simulink model "HANcoder_E407_TTA_Group2"  (R2018b)
settings: Solver=FixedStepDiscrete  StartTime=0.0  StopTime=1  FixedStep=0.01  RelTol=1e-3
PreLoadFcn:
  | librarySetup
  | eval([bdroot,'_startup']) %Calling [modelName]_startup.m
values from neighbouring files (symbols this model uses):
  BackUp_Role = 4    [HANcoder_E407_TTA_Group2_startup.m]
  basic_cycle_duration_bc0 = TM_Reset_Board   + COMP_duration    (= 550)    [HANcoder_E407_TTA_Group2_startup.m]    (also in HANcoder_E407_TTA_Template_startup.m = 212)
  basic_cycle_duration_bc1 = TM_Reset_Var_bc1 + COMP_duration    (= 610)    [HANcoder_E407_TTA_Group2_startup.m]    (also in HANcoder_E407_TTA_Template_startup.m = 212)
  board1_online = Simulink.Parameter    [HANcoder_E407_TTA_Group2_startup.m]
  board2_online = Simulink.Parameter    [HANcoder_E407_TTA_Group2_startup.m]
  board3_online = Simulink.Parameter    [HANcoder_E407_TTA_Group2_startup.m]
  board4_online = Simulink.Parameter    [HANcoder_E407_TTA_Group2_startup.m]
  comm_delay_estimation1 = round(comm_delay_measured1*hardware_granularity/frequency_IRQ)    [HANcoder_E407_TTA_Group2_startup.m]    (also in HANcoder_E407_TTA_Template_startup.m)
  comm_delay_estimation2 = round(comm_delay_measured2*hardware_granularity/frequency_IRQ)    [HANcoder_E407_TTA_Group2_startup.m]    (also in HANcoder_E407_TTA_Template_startup.m)
  COMM_Period = 50    [HANcoder_E407_TTA_Group2_startup.m]    (also in HANcoder_E407_TTA_Template_startup.m = 40)
  COMM_Phase1 = Simulink.Parameter    [HANcoder_E407_TTA_Group2_startup.m]    (also in HANcoder_E407_TTA_Template_startup.m)
  COMM_Phase2 = Simulink.Parameter    [HANcoder_E407_TTA_Group2_startup.m]    (also in HANcoder_E407_TTA_Template_startup.m)
  COMM_Phase_init1 = Simulink.Parameter    [HANcoder_E407_TTA_Group2_startup.m]    (also in HANcoder_E407_TTA_Template_startup.m)
  COMM_Phase_init2 = Simulink.Parameter    [HANcoder_E407_TTA_Group2_startup.m]    (also in HANcoder_E407_TTA_Template_startup.m)
  COMP_duration = 20    [HANcoder_E407_TTA_Group2_startup.m]    (also in HANcoder_E407_TTA_Template_startup.m = 4)
  Controller1_Board = 1    [HANcoder_E407_TTA_Group2_startup.m]    (also in HANcoder_E407_TTA_Template_startup.m)
  Controller2_Board = 2    [HANcoder_E407_TTA_Group2_startup.m]    (also in HANcoder_E407_TTA_Template_startup.m)
  Controller3_Board = 3    [HANcoder_E407_TTA_Group2_startup.m]    (also in HANcoder_E407_TTA_Template_startup.m)
  Controller4_Board = 4    [HANcoder_E407_TTA_Group2_startup.m]
  delta_a_set = Simulink.Parameter    [HANcoder_E407_TTA_Group2_startup.m]
  delta_f_set = Simulink.Parameter    [HANcoder_E407_TTA_Group2_startup.m]
  delta_max = 1    [HANcoder_E407_TTA_Group2_startup.m]
  delta_min = -1    [HANcoder_E407_TTA_Group2_startup.m]
  delta_precision = 6    [HANcoder_E407_TTA_Group2_startup.m]
  e_width = 0.1    [HANcoder_E407_TTA_Group2_startup.m]
  ErrorLog_ID = 31    [HANcoder_E407_TTA_Group2_startup.m]
  frequency_IRQ = 100    [HANcoder_E407_TTA_Group2_startup.m]    (also in HANcoder_E407_TTA_Template_startup.m)
  HANtuneOverride = Simulink.Parameter    [HANcoder_E407_TTA_Group2_startup.m]    (also in HANcoder_E407_TTA_Template_startup.m)
  hardware_granularity = 1000000    [HANcoder_E407_TTA_Group2_startup.m]    (also in HANcoder_E407_TTA_Template_startup.m)
  I_a = 2.25    [HANcoder_E407_TTA_Group2_startup.m]
  I_f = 2.25    [HANcoder_E407_TTA_Group2_startup.m]
  idle_time_init = basic_cycle_duration_bc0 + basic_cycle_duration_bc1    (= 1160)    [HANcoder_E407_TTA_Group2_startup.m]    (also in HANcoder_E407_TTA_Template_startup.m = 424)
  Input_Gen_Board = 5    [HANcoder_E407_TTA_Group2_startup.m]
  LA_Clock_Gr = 1    [HANcoder_E407_TTA_Group2_startup.m]    (also in HANcoder_E407_TTA_Template_startup.m)
  LA_COMM_dly = 1    [HANcoder_E407_TTA_Group2_startup.m]    (also in HANcoder_E407_TTA_Template_startup.m)
  LA_COMM_Err = 1    [HANcoder_E407_TTA_Group2_startup.m]    (also in HANcoder_E407_TTA_Template_startup.m)
  LA_E_Desync = 1    [HANcoder_E407_TTA_Group2_startup.m]    (also in HANcoder_E407_TTA_Template_startup.m)
  LA_MEX_Flag = 1    [HANcoder_E407_TTA_Group2_startup.m]    (also in HANcoder_E407_TTA_Template_startup.m)
  LA_Task_Act = 1    [HANcoder_E407_TTA_Group2_startup.m]    (also in HANcoder_E407_TTA_Template_startup.m)
  m_v = 100.0    (= 100)    [HANcoder_E407_TTA_Group2_startup.m]
  Master_Role = 1    [HANcoder_E407_TTA_Group2_startup.m]    (also in HANcoder_E407_TTA_Template_startup.m)
  matrix_cycle_duration = basic_cycle_duration_bc0 + basic_cycle_duration_bc1    (= 1160)    [HANcoder_E407_TTA_Group2_startup.m]    (also in HANcoder_E407_TTA_Template_startup.m = 424)
  matrix_rows = 2    [HANcoder_E407_TTA_Group2_startup.m]    (also in HANcoder_E407_TTA_Template_startup.m)
  max_desync = 15    [HANcoder_E407_TTA_Group2_startup.m]    (also in HANcoder_E407_TTA_Template_startup.m)
  max_num_msgs_CAN1 = 2^Tx_bit_number-1    (= 7)    [HANcoder_E407_TTA_Group2_startup.m]    (also in HANcoder_E407_TTA_Template_startup.m)
  max_num_msgs_CAN2 = max_num_msgs_CAN1    (= 7)    [HANcoder_E407_TTA_Group2_startup.m]    (also in HANcoder_E407_TTA_Template_startup.m)
  min_desync = (-1)*max_desync    (= -15)    [HANcoder_E407_TTA_Group2_startup.m]    (also in HANcoder_E407_TTA_Template_startup.m)
  OutControl1_ID = 23    [HANcoder_E407_TTA_Group2_startup.m]    (also in HANcoder_E407_TTA_Template_startup.m)
  OutControl2_ID = 24    [HANcoder_E407_TTA_Group2_startup.m]    (also in HANcoder_E407_TTA_Template_startup.m)
  OutEmulator_ID = 25    [HANcoder_E407_TTA_Group2_startup.m]    (also in HANcoder_E407_TTA_Template_startup.m)
  R_al = 0.10    (= 0.1)    [HANcoder_E407_TTA_Group2_startup.m]
  R_ar = 0.10    (= 0.1)    [HANcoder_E407_TTA_Group2_startup.m]
  R_fl = 0.10    (= 0.1)    [HANcoder_E407_TTA_Group2_startup.m]
  R_fr = 0.10    (= 0.1)    [HANcoder_E407_TTA_Group2_startup.m]
  script_run = Simulink.Parameter    [HANcoder_E407_TTA_Group2_startup.m]    (also in HANcoder_E407_TTA_Template_startup.m)
  SensorValues_ID = 22    [HANcoder_E407_TTA_Group2_startup.m]    (also in HANcoder_E407_TTA_Template_startup.m)
  SetValues_ID = 21    [HANcoder_E407_TTA_Group2_startup.m]    (also in HANcoder_E407_TTA_Template_startup.m)
  Slave_Role = 3    [HANcoder_E407_TTA_Group2_startup.m]    (also in HANcoder_E407_TTA_Template_startup.m = 2)
  speed_k_d = Simulink.Parameter    [HANcoder_E407_TTA_Group2_startup.m]
  speed_k_i = Simulink.Parameter    [HANcoder_E407_TTA_Group2_startup.m]
  speed_k_p = Simulink.Parameter    [HANcoder_E407_TTA_Group2_startup.m]
  speed_max = 10    [HANcoder_E407_TTA_Group2_startup.m]
  speed_min = -10    [HANcoder_E407_TTA_Group2_startup.m]
  speed_precision = 3    [HANcoder_E407_TTA_Group2_startup.m]
  Sync_ID = 1    [HANcoder_E407_TTA_Group2_startup.m]    (also in HANcoder_E407_TTA_Template_startup.m)
  tau_max = 5    [HANcoder_E407_TTA_Group2_startup.m]
  tau_min = -5    [HANcoder_E407_TTA_Group2_startup.m]
  tau_range = abs(tau_max) + abs(tau_min)    [HANcoder_E407_TTA_Group2_startup.m]
  theta_max = (speed_max/R_fr)*matrix_cycle_duration*frequency_IRQ/hardware_granularity    (= 11.6)    [HANcoder_E407_TTA_Group2_startup.m]
  theta_min = (-1)*theta_max    (= -11.6)    [HANcoder_E407_TTA_Group2_startup.m]
  theta_precision = 7-(fix(log2(theta_max))+1)    [HANcoder_E407_TTA_Group2_startup.m]
  Tl_a = 0.6    [HANcoder_E407_TTA_Group2_startup.m]
  Tl_f = 0.6    [HANcoder_E407_TTA_Group2_startup.m]
  TM_bc0_1 = basic_cycle_start    (= 0)    [HANcoder_E407_TTA_Group2_startup.m]
  TM_bc0_10 = TM_bc0_9 + COMP_duration    (= 270)    [HANcoder_E407_TTA_Group2_startup.m]
  TM_bc0_11 = TM_bc0_10 + COMP_duration    (= 290)    [HANcoder_E407_TTA_Group2_startup.m]
  TM_bc0_12 = TM_bc0_11  + COMM_duration    (= 340)    [HANcoder_E407_TTA_Group2_startup.m]
  TM_bc0_13 = TM_bc0_12 + COMP_duration    (= 360)    [HANcoder_E407_TTA_Group2_startup.m]
  TM_bc0_14 = TM_bc0_13 + COMP_duration    (= 380)    [HANcoder_E407_TTA_Group2_startup.m]
  TM_bc0_15 = TM_bc0_14  + COMM_duration    (= 430)    [HANcoder_E407_TTA_Group2_startup.m]
  TM_bc0_16 = TM_bc0_15 + COMP_duration    (= 450)    [HANcoder_E407_TTA_Group2_startup.m]
  TM_bc0_17 = TM_bc0_16 + COMP_duration    (= 470)    [HANcoder_E407_TTA_Group2_startup.m]
  TM_bc0_18 = TM_bc0_17 + COMP_duration    (= 490)    [HANcoder_E407_TTA_Group2_startup.m]
  TM_bc0_2 = TM_bc0_1   + COMM_duration    (= 50)    [HANcoder_E407_TTA_Group2_startup.m]
  TM_bc0_3 = TM_bc0_2  + COMP_duration    (= 70)    [HANcoder_E407_TTA_Group2_startup.m]
  TM_bc0_3_2 = TM_bc0_3   + 2    (= 72)    [HANcoder_E407_TTA_Group2_startup.m]
  TM_bc0_4 = TM_bc0_3   + COMP_duration    (= 90)    [HANcoder_E407_TTA_Group2_startup.m]
  TM_bc0_4_2 = TM_bc0_4    + 2    (= 92)    [HANcoder_E407_TTA_Group2_startup.m]
  TM_bc0_5 = TM_bc0_4    + COMP_duration    (= 110)    [HANcoder_E407_TTA_Group2_startup.m]
  TM_bc0_6 = TM_bc0_5  + COMM_duration    (= 160)    [HANcoder_E407_TTA_Group2_startup.m]
  TM_bc0_7 = TM_bc0_6 + COMP_duration    (= 180)    [HANcoder_E407_TTA_Group2_startup.m]
  TM_bc0_8 = TM_bc0_7 + COMP_duration    (= 200)    [HANcoder_E407_TTA_Group2_startup.m]
  TM_bc0_9 = TM_bc0_8  + COMM_duration    (= 250)    [HANcoder_E407_TTA_Group2_startup.m]
  TM_bc0_9_2 = TM_bc0_9 + 2    (= 252)    [HANcoder_E407_TTA_Group2_startup.m]
  TM_bc1_18 = TM_Check_Output_Emulator + COMP_duration    (= 520)    [HANcoder_E407_TTA_Group2_startup.m]
  TM_bc1_19 = TM_bc1_18 + COMM_duration    (= 570)    [HANcoder_E407_TTA_Group2_startup.m]
  TM_bc1_19_2 = TM_bc1_19 + 2    (= 572)    [HANcoder_E407_TTA_Group2_startup.m]
  TM_Check_Output_Control1 = TM_COMM_Output_Control1 + COMP_duration    (= 340)    [HANcoder_E407_TTA_Group2_startup.m]
  TM_Check_Output_Control2 = TM_COMM_Output_Control2 + COMM_duration    (= 410)    [HANcoder_E407_TTA_Group2_startup.m]
  TM_Check_Output_Emulator = TM_COMM_Output_Emulator + COMM_duration    (= 500)    [HANcoder_E407_TTA_Group2_startup.m]
  TM_Check_Output_Emulator_2 = TM_Check_Output_Emulator + 2    (= 502)    [HANcoder_E407_TTA_Group2_startup.m]
  TM_Check_Sensor_Values = TM_COMM_Sensor_Values + COMM_duration    (= 210)    [HANcoder_E407_TTA_Group2_startup.m]
  TM_Check_Sensor_Values_2 = TM_Check_Sensor_Values + 2    (= 212)    [HANcoder_E407_TTA_Group2_startup.m]
  TM_Check_Set_Values = TM_COMM_Set_Values + COMM_duration    (= 140)    [HANcoder_E407_TTA_Group2_startup.m]
  TM_Check_Set_Values_2 = TM_Check_Set_Values + 2    (= 142)    [HANcoder_E407_TTA_Group2_startup.m]
  TM_COMM_Output_Control1 = TM_Velocity + COMM_duration    (= 320)    [HANcoder_E407_TTA_Group2_startup.m]
  TM_COMM_Output_Control2 = TM_Check_Output_Control1 + COMP_duration    (= 360)    [HANcoder_E407_TTA_Group2_startup.m]
  TM_COMM_Output_Emulator = TM_TMR + COMP_duration    (= 450)    [HANcoder_E407_TTA_Group2_startup.m]
  TM_COMM_Sensor_Values = TM_Check_Set_Values + COMP_duration    (= 160)    [HANcoder_E407_TTA_Group2_startup.m]
  TM_COMM_Set_Values = TM_bc0_3 + COMP_duration    (= 90)    [HANcoder_E407_TTA_Group2_startup.m]
  TM_COMM_Sync = basic_cycle_start    (= 0)    [HANcoder_E407_TTA_Group2_startup.m]    (also in HANcoder_E407_TTA_Template_startup.m)
  TM_Data_bc0 = TM_COMM_Sync    (= 0)    [HANcoder_E407_TTA_Group2_startup.m]    (also in HANcoder_E407_TTA_Template_startup.m)
  TM_Data_bc1 = TM_Data_bc0(1:4)    [HANcoder_E407_TTA_Group2_startup.m]    (also in HANcoder_E407_TTA_Template_startup.m)
  TM_Reset_Board = TM_Reset_Var   + COMP_duration    (= 530)    [HANcoder_E407_TTA_Group2_startup.m]    (also in HANcoder_E407_TTA_Template_startup.m = 208)
  TM_Reset_Var = TM_bc0_18  + COMP_duration    (= 510)    [HANcoder_E407_TTA_Group2_startup.m]    (also in HANcoder_E407_TTA_Template_startup.m = 204)
  TM_Reset_Var_bc1 = TM_bc1_19 + COMP_duration    (= 590)    [HANcoder_E407_TTA_Group2_startup.m]    (also in HANcoder_E407_TTA_Template_startup.m = 200)
  TM_Reset_Var_bc1_2 = TM_Reset_Var_bc1 + 2    (= 592)    [HANcoder_E407_TTA_Group2_startup.m]    (also in HANcoder_E407_TTA_Template_startup.m = 202)
  TM_Steer = TM_Check_Sensor_Values + COMP_duration    (= 230)    [HANcoder_E407_TTA_Group2_startup.m]
  TM_TMR = TM_Check_Output_Control2 + COMP_duration    (= 430)    [HANcoder_E407_TTA_Group2_startup.m]
  TM_TMR_2 = TM_TMR + 1    (= 431)    [HANcoder_E407_TTA_Group2_startup.m]
  ... (+19 more)
undefined symbols (not defined in the file or in its folder): A0, A1, A2, A3, A4, CON2, CON4, D10, D12, D13, D8, D9
libraries: hdlsllib x340, HANcoder_STM32_Target x28, simulink x5, simulink_extras x1
(part 6 of 36)

== system HANcoder_E407_TTA_Group2/HANcoder STM32 Target - E407-STM32 algorithm/TTA CAN System/CAN1 Recieve/RxID_CAN/SetValues_ID_CAN/CAN receive1 ==
  In1 : Inport
  Enabled Subsystem : Subsystem  TreatAsAtomicUnit=on
  S-Function : M-S-Function  FunctionName=sfcn_can_receive  Parameters=tsamp, canBus, outputNumber, dataType, byteOrder
  Out1 : Outport
  Out2 : Outport  Port=2
  Out3 : Outport  Port=3
  Out4 : Outport  Port=4
  Out5 : Outport  Port=5
  Out6 : Outport  Port=6
  Out7 : Outport  Port=7
  Out8 : Outport  Port=8
  Out9 : Outport  Port=9
  wires:
  S-Function/9 -> Enabled Subsystem/8(In8)
  S-Function/4 -> Enabled Subsystem/3(In3)
  S-Function/5 -> Enabled Subsystem/4(In4)
  S-Function/8 -> Enabled Subsystem/7(In7)
  S-Function/7 -> Enabled Subsystem/6(In6)
  S-Function/6 -> Enabled Subsystem/5(In5)
  Enabled Subsystem/8(Out8) -> Out9/1
  Enabled Subsystem/7(Out7) -> Out8/1
  Enabled Subsystem/6(Out6) -> Out7/1
  Enabled Subsystem/5(Out5) -> Out6/1
  Enabled Subsystem/4(Out4) -> Out5/1
  Enabled Subsystem/3(Out3) -> Out4/1
  Enabled Subsystem/2(Out2) -> Out3/1
  Enabled Subsystem/1(Out1) -> Out2/1
  S-Function/3 -> Enabled Subsystem/2(In2)
  S-Function/2 -> Enabled Subsystem/1(In1)
  S-Function/1 -> Out1/1, Enabled Subsystem/Enable
  In1/1 -> S-Function/1

== system HANcoder_E407_TTA_Group2/HANcoder STM32 Target - E407-STM32 algorithm/TTA CAN System/CAN1 Recieve/RxID_CAN/Sync_ID_CAN/CAN receive1 ==
  In1 : Inport
  Enabled Subsystem : Subsystem  TreatAsAtomicUnit=on
  S-Function : M-S-Function  FunctionName=sfcn_can_receive  Parameters=tsamp, canBus, outputNumber, dataType, byteOrder
  Out1 : Outport
  Out2 : Outport  Port=2
  Out3 : Outport  Port=3
  Out4 : Outport  Port=4
  Out5 : Outport  Port=5
  Out6 : Outport  Port=6
  Out7 : Outport  Port=7
  Out8 : Outport  Port=8
  Out9 : Outport  Port=9
  wires:
  S-Function/9 -> Enabled Subsystem/8(In8)
  S-Function/4 -> Enabled Subsystem/3(In3)
  S-Function/5 -> Enabled Subsystem/4(In4)
  S-Function/8 -> Enabled Subsystem/7(In7)
  S-Function/7 -> Enabled Subsystem/6(In6)
  S-Function/6 -> Enabled Subsystem/5(In5)
  Enabled Subsystem/8(Out8) -> Out9/1
  Enabled Subsystem/7(Out7) -> Out8/1
  Enabled Subsystem/6(Out6) -> Out7/1
  Enabled Subsystem/5(Out5) -> Out6/1
  Enabled Subsystem/4(Out4) -> Out5/1
  Enabled Subsystem/3(Out3) -> Out4/1
  Enabled Subsystem/2(Out2) -> Out3/1
  Enabled Subsystem/1(Out1) -> Out2/1
  S-Function/3 -> Enabled Subsystem/2(In2)
  S-Function/2 -> Enabled Subsystem/1(In1)
  S-Function/1 -> Out1/1, Enabled Subsystem/Enable
  In1/1 -> S-Function/1

== system HANcoder_E407_TTA_Group2/HANcoder STM32 Target - E407-STM32 algorithm/TTA CAN System/CAN1 Recieve/RxID_CAN/Vote1_ID_CAN/CAN receive1 ==
  In1 : Inport
  Enabled Subsystem : Subsystem  TreatAsAtomicUnit=on
  S-Function : M-S-Function  FunctionName=sfcn_can_receive  Parameters=tsamp, canBus, outputNumber, dataType, byteOrder
  Out1 : Outport
  Out2 : Outport  Port=2
  Out3 : Outport  Port=3
  Out4 : Outport  Port=4
  Out5 : Outport  Port=5
  Out6 : Outport  Port=6
  Out7 : Outport  Port=7
  Out8 : Outport  Port=8
  Out9 : Outport  Port=9
  wires:
  In1/1 -> S-Function/1
  S-Function/1 -> Enabled Subsystem/Enable, Out1/1
  S-Function/2 -> Enabled Subsystem/1(In1)
  S-Function/3 -> Enabled Subsystem/2(In2)
  Enabled Subsystem/1(Out1) -> Out2/1
  Enabled Subsystem/2(Out2) -> Out3/1
  Enabled Subsystem/3(Out3) -> Out4/1
  Enabled Subsystem/4(Out4) -> Out5/1
  Enabled Subsystem/5(Out5) -> Out6/1
  Enabled Subsystem/6(Out6) -> Out7/1
  Enabled Subsystem/7(Out7) -> Out8/1
  Enabled Subsystem/8(Out8) -> Out9/1
  S-Function/6 -> Enabled Subsystem/5(In5)
  S-Function/7 -> Enabled Subsystem/6(In6)
  S-Function/8 -> Enabled Subsystem/7(In7)
  S-Function/5 -> Enabled Subsystem/4(In4)
  S-Function/4 -> Enabled Subsystem/3(In3)
  S-Function/9 -> Enabled Subsystem/8(In8)

== system HANcoder_E407_TTA_Group2/HANcoder STM32 Target - E407-STM32 algorithm/TTA CAN System/CAN1 Recieve/RxID_CAN/Vote2_ID_CAN/CAN receive1 ==
  In1 : Inport
  Enabled Subsystem : Subsystem  TreatAsAtomicUnit=on
  S-Function : M-S-Function  FunctionName=sfcn_can_receive  Parameters=tsamp, canBus, outputNumber, dataType, byteOrder
  Out1 : Outport
  Out2 : Outport  Port=2
  Out3 : Outport  Port=3
  Out4 : Outport  Port=4
  Out5 : Outport  Port=5
  Out6 : Outport  Port=6
  Out7 : Outport  Port=7
  Out8 : Outport  Port=8
  Out9 : Outport  Port=9
  wires:
  In1/1 -> S-Function/1
  S-Function/1 -> Enabled Subsystem/Enable, Out1/1
  S-Function/2 -> Enabled Subsystem/1(In1)
  S-Function/3 -> Enabled Subsystem/2(In2)
  Enabled Subsystem/1(Out1) -> Out2/1
  Enabled Subsystem/2(Out2) -> Out3/1
  Enabled Subsystem/3(Out3) -> Out4/1
  Enabled Subsystem/4(Out4) -> Out5/1
  Enabled Subsystem/5(Out5) -> Out6/1
  Enabled Subsystem/6(Out6) -> Out7/1
  Enabled Subsystem/7(Out7) -> Out8/1
  Enabled Subsystem/8(Out8) -> Out9/1
  S-Function/6 -> Enabled Subsystem/5(In5)
  S-Function/7 -> Enabled Subsystem/6(In6)
  S-Function/8 -> Enabled Subsystem/7(In7)
  S-Function/5 -> Enabled Subsystem/4(In4)
  S-Function/4 -> Enabled Subsystem/3(In3)
  S-Function/9 -> Enabled Subsystem/8(In8)

== system HANcoder_E407_TTA_Group2/HANcoder STM32 Target - E407-STM32 algorithm/TTA CAN System/CAN1 Recieve/RxID_CAN/Vote3_ID_CAN/CAN receive1 ==
  In1 : Inport
  Enabled Subsystem : Subsystem  TreatAsAtomicUnit=on
  S-Function : M-S-Function  FunctionName=sfcn_can_receive  Parameters=tsamp, canBus, outputNumber, dataType, byteOrder
  Out1 : Outport
  Out2 : Outport  Port=2
  Out3 : Outport  Port=3
  Out4 : Outport  Port=4
  Out5 : Outport  Port=5
  Out6 : Outport  Port=6
  Out7 : Outport  Port=7
  Out8 : Outport  Port=8
  Out9 : Outport  Port=9
  wires:
  In1/1 -> S-Function/1
  S-Function/1 -> Enabled Subsystem/Enable, Out1/1
  S-Function/2 -> Enabled Subsystem/1(In1)
  S-Function/3 -> Enabled Subsystem/2(In2)
  Enabled Subsystem/1(Out1) -> Out2/1
  Enabled Subsystem/2(Out2) -> Out3/1
  Enabled Subsystem/3(Out3) -> Out4/1
  Enabled Subsystem/4(Out4) -> Out5/1
  Enabled Subsystem/5(Out5) -> Out6/1
  Enabled Subsystem/6(Out6) -> Out7/1
  Enabled Subsystem/7(Out7) -> Out8/1
  Enabled Subsystem/8(Out8) -> Out9/1
  S-Function/6 -> Enabled Subsystem/5(In5)
  S-Function/7 -> Enabled Subsystem/6(In6)
  S-Function/8 -> Enabled Subsystem/7(In7)
  S-Function/5 -> Enabled Subsystem/4(In4)
  S-Function/4 -> Enabled Subsystem/3(In3)
  S-Function/9 -> Enabled Subsystem/8(In8)

== system HANcoder_E407_TTA_Group2/HANcoder STM32 Target - E407-STM32 algorithm/TTA CAN System/CAN1 Recieve/RxID_CAN/Vote4_ID_CAN1/CAN receive1 ==
  In1 : Inport
  Enabled Subsystem : Subsystem  TreatAsAtomicUnit=on
  S-Function : M-S-Function  FunctionName=sfcn_can_receive  Parameters=tsamp, canBus, outputNumber, dataType, byteOrder
  Out1 : Outport
  Out2 : Outport  Port=2
  Out3 : Outport  Port=3
  Out4 : Outport  Port=4
  Out5 : Outport  Port=5
  Out6 : Outport  Port=6
  Out7 : Outport  Port=7
  Out8 : Outport  Port=8
  Out9 : Outport  Port=9
  wires:
  In1/1 -> S-Function/1
  S-Function/1 -> Enabled Subsystem/Enable, Out1/1
  S-Function/2 -> Enabled Subsystem/1(In1)
  S-Function/3 -> Enabled Subsystem/2(In2)
  Enabled Subsystem/1(Out1) -> Out2/1
  Enabled Subsystem/2(Out2) -> Out3/1
  Enabled Subsystem/3(Out3) -> Out4/1
  Enabled Subsystem/4(Out4) -> Out5/1
  Enabled Subsystem/5(Out5) -> Out6/1
  Enabled Subsystem/6(Out6) -> Out7/1
  Enabled Subsystem/7(Out7) -> Out8/1
  Enabled Subsystem/8(Out8) -> Out9/1
  S-Function/6 -> Enabled Subsystem/5(In5)
  S-Function/7 -> Enabled Subsystem/6(In6)
  S-Function/8 -> Enabled Subsystem/7(In7)
  S-Function/5 -> Enabled Subsystem/4(In4)
  S-Function/4 -> Enabled Subsystem/3(In3)
  S-Function/9 -> Enabled Subsystem/8(In8)

== system HANcoder_E407_TTA_Group2/HANcoder STM32 Target - E407-STM32 algorithm/TTA CAN System/CAN2 Recieve/RxID_CAN/OutControl1_ID_CAN/CAN receive1 ==
  In1 : Inport
  Enabled Subsystem : Subsystem  TreatAsAtomicUnit=on
  S-Function : M-S-Function  FunctionName=sfcn_can_receive  Parameters=tsamp, canBus, outputNumber, dataType, byteOrder
  Out1 : Outport
  Out2 : Outport  Port=2
  Out3 : Outport  Port=3
  Out4 : Outport  Port=4
  Out5 : Outport  Port=5
  Out6 : Outport  Port=6
  Out7 : Outport  Port=7
  Out8 : Outport  Port=8
  Out9 : Outport  Port=9
  wires:
  S-Function/9 -> Enabled Subsystem/8(In8)
  S-Function/4 -> Enabled Subsystem/3(In3)
  S-Function/5 -> Enabled Subsystem/4(In4)
  S-Function/8 -> Enabled Subsystem/7(In7)
  S-Function/7 -> Enabled Subsystem/6(In6)
  S-Function/6 -> Enabled Subsystem/5(In5)
  Enabled Subsystem/8(Out8) -> Out9/1
  Enabled Subsystem/7(Out7) -> Out8/1
  Enabled Subsystem/6(Out6) -> Out7/1
  Enabled Subsystem/5(Out5) -> Out6/1
  Enabled Subsystem/4(Out4) -> Out5/1
  Enabled Subsystem/3(Out3) -> Out4/1
  Enabled Subsystem/2(Out2) -> Out3/1
  Enabled Subsystem/1(Out1) -> Out2/1
  S-Function/3 -> Enabled Subsystem/2(In2)
  S-Function/2 -> Enabled Subsystem/1(In1)
  S-Function/1 -> Out1/1, Enabled Subsystem/Enable
  In1/1 -> S-Function/1

== system HANcoder_E407_TTA_Group2/HANcoder STM32 Target - E407-STM32 algorithm/TTA CAN System/CAN2 Recieve/RxID_CAN/OutControl2_ID_CAN/CAN receive1 ==
  In1 : Inport
  Enabled Subsystem : Subsystem  TreatAsAtomicUnit=on
  S-Function : M-S-Function  FunctionName=sfcn_can_receive  Parameters=tsamp, canBus, outputNumber, dataType, byteOrder
  Out1 : Outport
  Out2 : Outport  Port=2
  Out3 : Outport  Port=3
  Out4 : Outport  Port=4
  Out5 : Outport  Port=5
  Out6 : Outport  Port=6
  Out7 : Outport  Port=7
  Out8 : Outport  Port=8
  Out9 : Outport  Port=9
  wires:
  In1/1 -> S-Function/1
  S-Function/1 -> Enabled Subsystem/Enable, Out1/1
  S-Function/2 -> Enabled Subsystem/1(In1)
  S-Function/3 -> Enabled Subsystem/2(In2)
  Enabled Subsystem/1(Out1) -> Out2/1
  Enabled Subsystem/2(Out2) -> Out3/1
  Enabled Subsystem/3(Out3) -> Out4/1
  Enabled Subsystem/4(Out4) -> Out5/1
  Enabled Subsystem/5(Out5) -> Out6/1
  Enabled Subsystem/6(Out6) -> Out7/1
  Enabled Subsystem/7(Out7) -> Out8/1
  Enabled Subsystem/8(Out8) -> Out9/1
  S-Function/6 -> Enabled Subsystem/5(In5)
  S-Function/7 -> Enabled Subsystem/6(In6)
  S-Function/8 -> Enabled Subsystem/7(In7)
  S-Function/5 -> Enabled Subsystem/4(In4)
  S-Function/4 -> Enabled Subsystem/3(In3)
  S-Function/9 -> Enabled Subsystem/8(In8)

== system HANcoder_E407_TTA_Group2/HANcoder STM32 Target - E407-STM32 algorithm/TTA CAN System/CAN2 Recieve/RxID_CAN/OutEmulator_ID_CAN/CAN receive1 ==
  In1 : Inport
  Enabled Subsystem : Subsystem  TreatAsAtomicUnit=on
  S-Function : M-S-Function  FunctionName=sfcn_can_receive  Parameters=tsamp, canBus, outputNumber, dataType, byteOrder
  Out1 : Outport
  Out2 : Outport  Port=2
  Out3 : Outport  Port=3
  Out4 : Outport  Port=4
  Out5 : Outport  Port=5
  Out6 : Outport  Port=6
  Out7 : Outport  Port=7
  Out8 : Outport  Port=8
  Out9 : Outport  Port=9
  wires:
  S-Function/9 -> Enabled Subsystem/8(In8)
  S-Function/4 -> Enabled Subsystem/3(In3)
  S-Function/5 -> Enabled Subsystem/4(In4)
  S-Function/8 -> Enabled Subsystem/7(In7)
  S-Function/7 -> Enabled Subsystem/6(In6)
  S-Function/6 -> Enabled Subsystem/5(In5)
  Enabled Subsystem/8(Out8) -> Out9/1
  Enabled Subsystem/7(Out7) -> Out8/1
  Enabled Subsystem/6(Out6) -> Out7/1
  Enabled Subsystem/5(Out5) -> Out6/1
  Enabled Subsystem/4(Out4) -> Out5/1
  Enabled Subsystem/3(Out3) -> Out4/1
  Enabled Subsystem/2(Out2) -> Out3/1
  Enabled Subsystem/1(Out1) -> Out2/1
  S-Function/3 -> Enabled Subsystem/2(In2)
  S-Function/2 -> Enabled Subsystem/1(In1)
  S-Function/1 -> Out1/1, Enabled Subsystem/Enable
  In1/1 -> S-Function/1

== system HANcoder_E407_TTA_Group2/HANcoder STM32 Target - E407-STM32 algorithm/TTA CAN System/CAN2 Recieve/RxID_CAN/OutEmulator_ID_CAN1/CAN receive1 ==
  In1 : Inport
  Enabled Subsystem : Subsystem  TreatAsAtomicUnit=on
  S-Function : M-S-Function  FunctionName=sfcn_can_receive  Parameters=tsamp, canBus, outputNumber, dataType, byteOrder
  Out1 : Outport
  Out2 : Outport  Port=2
  Out3 : Outport  Port=3
  Out4 : Outport  Port=4
  Out5 : Outport  Port=5
  Out6 : Outport  Port=6
  Out7 : Outport  Port=7
  Out8 : Outport  Port=8
  Out9 : Outport  Port=9
  wires:
  S-Function/9 -> Enabled Subsystem/8(In8)
  S-Function/4 -> Enabled Subsystem/3(In3)
  S-Function/5 -> Enabled Subsystem/4(In4)
  S-Function/8 -> Enabled Subsystem/7(In7)
  S-Function/7 -> Enabled Subsystem/6(In6)
  S-Function/6 -> Enabled Subsystem/5(In5)
  Enabled Subsystem/8(Out8) -> Out9/1
  Enabled Subsystem/7(Out7) -> Out8/1
  Enabled Subsystem/6(Out6) -> Out7/1
  Enabled Subsystem/5(Out5) -> Out6/1
  Enabled Subsystem/4(Out4) -> Out5/1
  Enabled Subsystem/3(Out3) -> Out4/1
  Enabled Subsystem/2(Out2) -> Out3/1
  Enabled Subsystem/1(Out1) -> Out2/1
  S-Function/3 -> Enabled Subsystem/2(In2)
  S-Function/2 -> Enabled Subsystem/1(In1)
  S-Function/1 -> Out1/1, Enabled Subsystem/Enable
  In1/1 -> S-Function/1

== system HANcoder_E407_TTA_Group2/HANcoder STM32 Target - E407-STM32 algorithm/TTA CAN System/CAN2 Recieve/RxID_CAN/SensorValues_ID_CAN/CAN receive1 ==
  In1 : Inport
  Enabled Subsystem : Subsystem  TreatAsAtomicUnit=on
  S-Function : M-S-Function  FunctionName=sfcn_can_receive  Parameters=tsamp, canBus, outputNumber, dataType, byteOrder
  Out1 : Outport
  Out2 : Outport  Port=2
  Out3 : Outport  Port=3
  Out4 : Outport  Port=4
  Out5 : Outport  Port=5
  Out6 : Outport  Port=6
  Out7 : Outport  Port=7
  Out8 : Outport  Port=8
  Out9 : Outport  Port=9
  wires:
  In1/1 -> S-Function/1
  S-Function/1 -> Enabled Subsystem/Enable, Out1/1
  S-Function/2 -> Enabled Subsystem/1(In1)
  S-Function/3 -> Enabled Subsystem/2(In2)
  Enabled Subsystem/1(Out1) -> Out2/1
  Enabled Subsystem/2(Out2) -> Out3/1
  Enabled Subsystem/3(Out3) -> Out4/1
  Enabled Subsystem/4(Out4) -> Out5/1
  Enabled Subsystem/5(Out5) -> Out6/1
  Enabled Subsystem/6(Out6) -> Out7/1
  Enabled Subsystem/7(Out7) -> Out8/1
  Enabled Subsystem/8(Out8) -> Out9/1
  S-Function/6 -> Enabled Subsystem/5(In5)
  S-Function/7 -> Enabled Subsystem/6(In6)
  S-Function/8 -> Enabled Subsystem/7(In7)
  S-Function/5 -> Enabled Subsystem/4(In4)
  S-Function/4 -> Enabled Subsystem/3(In3)
  S-Function/9 -> Enabled Subsystem/8(In8)

== system HANcoder_E407_TTA_Group2/HANcoder STM32 Target - E407-STM32 algorithm/TTA CAN System/CAN2 Recieve/RxID_CAN/SetValues_ID_CAN/CAN receive1 ==
  In1 : Inport
  Enabled Subsystem : Subsystem  TreatAsAtomicUnit=on
  S-Function : M-S-Function  FunctionName=sfcn_can_receive  Parameters=tsamp, canBus, outputNumber, dataType, byteOrder
  Out1 : Outport
  Out2 : Outport  Port=2
  Out3 : Outport  Port=3
  Out4 : Outport  Port=4
  Out5 : Outport  Port=5
  Out6 : Outport  Port=6
  Out7 : Outport  Port=7
  Out8 : Outport  Port=8
  Out9 : Outport  Port=9
  wires:
  S-Function/9 -> Enabled Subsystem/8(In8)
  S-Function/4 -> Enabled Subsystem/3(In3)
  S-Function/5 -> Enabled Subsystem/4(In4)
  S-Function/8 -> Enabled Subsystem/7(In7)
  S-Function/7 -> Enabled Subsystem/6(In6)
  S-Function/6 -> Enabled Subsystem/5(In5)
  Enabled Subsystem/8(Out8) -> Out9/1
  Enabled Subsystem/7(Out7) -> Out8/1
  Enabled Subsystem/6(Out6) -> Out7/1
  Enabled Subsystem/5(Out5) -> Out6/1
  Enabled Subsystem/4(Out4) -> Out5/1
  Enabled Subsystem/3(Out3) -> Out4/1
  Enabled Subsystem/2(Out2) -> Out3/1
  Enabled Subsystem/1(Out1) -> Out2/1
  S-Function/3 -> Enabled Subsystem/2(In2)
  S-Function/2 -> Enabled Subsystem/1(In1)
  S-Function/1 -> Out1/1, Enabled Subsystem/Enable
  In1/1 -> S-Function/1

== system HANcoder_E407_TTA_Group2/HANcoder STM32 Target - E407-STM32 algorithm/TTA CAN System/CAN2 Recieve/RxID_CAN/Sync_ID_CAN/CAN receive1 ==
  In1 : Inport
  Enabled Subsystem : Subsystem  TreatAsAtomicUnit=on
  S-Function : M-S-Function  FunctionName=sfcn_can_receive  Parameters=tsamp, canBus, outputNumber, dataType, byteOrder
  Out1 : Outport
  Out2 : Outport  Port=2
  Out3 : Outport  Port=3
  Out4 : Outport  Port=4
  Out5 : Outport  Port=5
  Out6 : Outport  Port=6
  Out7 : Outport  Port=7
  Out8 : Outport  Port=8
  Out9 : Outport  Port=9
  wires:
  S-Function/9 -> Enabled Subsystem/8(In8)
  S-Function/4 -> Enabled Subsystem/3(In3)
  S-Function/5 -> Enabled Subsystem/4(In4)
  S-Function/8 -> Enabled Subsystem/7(In7)
  S-Function/7 -> Enabled Subsystem/6(In6)
  S-Function/6 -> Enabled Subsystem/5(In5)
  Enabled Subsystem/8(Out8) -> Out9/1
  Enabled Subsystem/7(Out7) -> Out8/1
  Enabled Subsystem/6(Out6) -> Out7/1
  Enabled Subsystem/5(Out5) -> Out6/1
  Enabled Subsystem/4(Out4) -> Out5/1
  Enabled Subsystem/3(Out3) -> Out4/1
  Enabled Subsystem/2(Out2) -> Out3/1
  Enabled Subsystem/1(Out1) -> Out2/1
  S-Function/3 -> Enabled Subsystem/2(In2)
  S-Function/2 -> Enabled Subsystem/1(In1)
  S-Function/1 -> Out1/1, Enabled Subsystem/Enable
  In1/1 -> S-Function/1

== system HANcoder_E407_TTA_Group2/HANcoder STM32 Target - E407-STM32 algorithm/TTA CAN System/CAN2 Recieve/RxID_CAN/Vote1_ID_CAN/CAN receive1 ==
  In1 : Inport
  Enabled Subsystem : Subsystem  TreatAsAtomicUnit=on
  S-Function : M-S-Function  FunctionName=sfcn_can_receive  Parameters=tsamp, canBus, outputNumber, dataType, byteOrder
  Out1 : Outport
  Out2 : Outport  Port=2
  Out3 : Outport  Port=3
  Out4 : Outport  Port=4
  Out5 : Outport  Port=5
  Out6 : Outport  Port=6
  Out7 : Outport  Port=7
  Out8 : Outport  Port=8
  Out9 : Outport  Port=9
  wires:
  In1/1 -> S-Function/1
  S-Function/1 -> Enabled Subsystem/Enable, Out1/1
  S-Function/2 -> Enabled Subsystem/1(In1)
  S-Function/3 -> Enabled Subsystem/2(In2)
  Enabled Subsystem/1(Out1) -> Out2/1
  Enabled Subsystem/2(Out2) -> Out3/1
  Enabled Subsystem/3(Out3) -> Out4/1
  Enabled Subsystem/4(Out4) -> Out5/1
  Enabled Subsystem/5(Out5) -> Out6/1
  Enabled Subsystem/6(Out6) -> Out7/1
  Enabled Subsystem/7(Out7) -> Out8/1
  Enabled Subsystem/8(Out8) -> Out9/1
  S-Function/6 -> Enabled Subsystem/5(In5)
  S-Function/7 -> Enabled Subsystem/6(In6)
  S-Function/8 -> Enabled Subsystem/7(In7)
  S-Function/5 -> Enabled Subsystem/4(In4)
  S-Function/4 -> Enabled Subsystem/3(In3)
  S-Function/9 -> Enabled Subsystem/8(In8)

== system HANcoder_E407_TTA_Group2/HANcoder STM32 Target - E407-STM32 algorithm/TTA CAN System/CAN2 Recieve/RxID_CAN/Vote2_ID_CAN/CAN receive1 ==
  In1 : Inport
  Enabled Subsystem : Subsystem  TreatAsAtomicUnit=on
  S-Function : M-S-Function  FunctionName=sfcn_can_receive  Parameters=tsamp, canBus, outputNumber, dataType, byteOrder
  Out1 : Outport
  Out2 : Outport  Port=2
  Out3 : Outport  Port=3
  Out4 : Outport  Port=4
  Out5 : Outport  Port=5
  Out6 : Outport  Port=6
  Out7 : Outport  Port=7
  Out8 : Outport  Port=8
  Out9 : Outport  Port=9
  wires:
  In1/1 -> S-Function/1
  S-Function/1 -> Enabled Subsystem/Enable, Out1/1
  S-Function/2 -> Enabled Subsystem/1(In1)
  S-Function/3 -> Enabled Subsystem/2(In2)
  Enabled Subsystem/1(Out1) -> Out2/1
  Enabled Subsystem/2(Out2) -> Out3/1
  Enabled Subsystem/3(Out3) -> Out4/1
  Enabled Subsystem/4(Out4) -> Out5/1
  Enabled Subsystem/5(Out5) -> Out6/1
  Enabled Subsystem/6(Out6) -> Out7/1
  Enabled Subsystem/7(Out7) -> Out8/1
  Enabled Subsystem/8(Out8) -> Out9/1
  S-Function/6 -> Enabled Subsystem/5(In5)
  S-Function/7 -> Enabled Subsystem/6(In6)
  S-Function/8 -> Enabled Subsystem/7(In7)
  S-Function/5 -> Enabled Subsystem/4(In4)
  S-Function/4 -> Enabled Subsystem/3(In3)
  S-Function/9 -> Enabled Subsystem/8(In8)

== system HANcoder_E407_TTA_Group2/HANcoder STM32 Target - E407-STM32 algorithm/TTA CAN System/CAN2 Recieve/RxID_CAN/Vote3_ID_CAN/CAN receive1 ==
  In1 : Inport
  Enabled Subsystem : Subsystem  TreatAsAtomicUnit=on
  S-Function : M-S-Function  FunctionName=sfcn_can_receive  Parameters=tsamp, canBus, outputNumber, dataType, byteOrder
  Out1 : Outport
  Out2 : Outport  Port=2
  Out3 : Outport  Port=3
  Out4 : Outport  Port=4
  Out5 : Outport  Port=5
  Out6 : Outport  Port=6
  Out7 : Outport  Port=7
  Out8 : Outport  Port=8
  Out9 : Outport  Port=9
  wires:
  In1/1 -> S-Function/1
  S-Function/1 -> Enabled Subsystem/Enable, Out1/1
  S-Function/2 -> Enabled Subsystem/1(In1)
  S-Function/3 -> Enabled Subsystem/2(In2)
  Enabled Subsystem/1(Out1) -> Out2/1
  Enabled Subsystem/2(Out2) -> Out3/1
  Enabled Subsystem/3(Out3) -> Out4/1
  Enabled Subsystem/4(Out4) -> Out5/1
  Enabled Subsystem/5(Out5) -> Out6/1
  Enabled Subsystem/6(Out6) -> Out7/1
  Enabled Subsystem/7(Out7) -> Out8/1
  Enabled Subsystem/8(Out8) -> Out9/1
  S-Function/6 -> Enabled Subsystem/5(In5)
  S-Function/7 -> Enabled Subsystem/6(In6)
  S-Function/8 -> Enabled Subsystem/7(In7)
  S-Function/5 -> Enabled Subsystem/4(In4)
  S-Function/4 -> Enabled Subsystem/3(In3)
  S-Function/9 -> Enabled Subsystem/8(In8)

== system HANcoder_E407_TTA_Group2/HANcoder STM32 Target - E407-STM32 algorithm/TTA CAN System/CAN2 Recieve/RxID_CAN/Vote3_ID_CAN1/CAN receive1 ==
  In1 : Inport
  Enabled Subsystem : Subsystem  TreatAsAtomicUnit=on
  S-Function : M-S-Function  FunctionName=sfcn_can_receive  Parameters=tsamp, canBus, outputNumber, dataType, byteOrder
  Out1 : Outport
  Out2 : Outport  Port=2
  Out3 : Outport  Port=3
  Out4 : Outport  Port=4
  Out5 : Outport  Port=5
  Out6 : Outport  Port=6
  Out7 : Outport  Port=7
  Out8 : Outport  Port=8
  Out9 : Outport  Port=9
  wires:
  In1/1 -> S-Function/1
  S-Function/1 -> Enabled Subsystem/Enable, Out1/1
  S-Function/2 -> Enabled Subsystem/1(In1)
  S-Function/3 -> Enabled Subsystem/2(In2)
  Enabled Subsystem/1(Out1) -> Out2/1
  Enabled Subsystem/2(Out2) -> Out3/1
  Enabled Subsystem/3(Out3) -> Out4/1
  Enabled Subsystem/4(Out4) -> Out5/1
  Enabled Subsystem/5(Out5) -> Out6/1
  Enabled Subsystem/6(Out6) -> Out7/1
  Enabled Subsystem/7(Out7) -> Out8/1
  Enabled Subsystem/8(Out8) -> Out9/1
  S-Function/6 -> Enabled Subsystem/5(In5)
  S-Function/7 -> Enabled Subsystem/6(In6)
  S-Function/8 -> Enabled Subsystem/7(In7)
  S-Function/5 -> Enabled Subsystem/4(In4)
  S-Function/4 -> Enabled Subsystem/3(In3)
  S-Function/9 -> Enabled Subsystem/8(In8)

== system HANcoder_E407_TTA_Group2/HANcoder STM32 Target - E407-STM32 algorithm/TTA CAN System/TTA System/Initialization/RoleID and Global Time init/Global Time Initialization Master ==
  note: Global Time Initialization
  Enable : EnablePort
  Board nr1 : Constant  Value=2
  Cast : DataTypeConversion  OutDataTypeStr=uint16
  Cast1 : DataTypeConversion  OutDataTypeStr=uint8
  Data Store Write : DataStoreWrite  DataStoreName=Local_Ticks
  Data Store Write1 : DataStoreWrite  DataStoreName=basic_cycle_count
  Data Store Write3 : DataStoreWrite  DataStoreName=Master_ID
  Start : Constant  Value=0
  wires:
  Board nr1/1 -> Data Store Write3/1
  Start/1 -> Cast1/1, Cast/1
  Cast/1 -> Data Store Write/1
  Cast1/1 -> Data Store Write1/1

== system HANcoder_E407_TTA_Group2/HANcoder STM32 Target - E407-STM32 algorithm/TTA CAN System/TTA System/Initialization/RoleID and Global Time init/Global Time Initialization Slave ==
  note: Sync has already been received, so we skip
      | the first comp tasks related to Update LT.
  note: Global Time Initialization
  note: Estimation of the Local Time when the message was sent
  Enable : EnablePort
  Bus Selector : BusSelector  OutputSignals=Buffer_1,Buffer_2,Buffer_3,Buffer_4,Buffer_5,Buffer_6,Buffer_7,Buffer_8
  Cast : DataTypeConversion  OutDataTypeStr=uint16
  Cast1 : DataTypeConversion  OutDataTypeStr=double
  Constant : Constant
  Constant1 : Constant  Value=COMM_Phase1
  Constant2 : Constant  Value=COMM_Phase2
  Constant3 : Constant  Value=TM_COMM_Sync
  Data Store Read : DataStoreRead  DataStoreName=New_Msg_Ready_CAN1
  Data Store Read1 : DataStoreRead  DataStoreName=Msg_Rx_CAN1
  Data Store Read2 : DataStoreRead  DataStoreName=Msg_Rx_CAN2
  Data Store Write1 : DataStoreWrite  DataStoreName=Local_Ticks
  Data Store Write2 : DataStoreWrite  DataStoreName=basic_cycle_count
  Data Store Write3 : DataStoreWrite  DataStoreName=Master_ID
  Data Store Write4 : DataStoreWrite  Priority=10  DataStoreName=BC0_Sync_processed
  Equal : RelationalOperator  Operator===  OutDataTypeStr=boolean  RndMeth=Simplest
  Multiply : Product
  Multiply1 : Product
  "SET1 " : Constant  Priority=9  OutDataTypeStr=boolean
  Sum : Sum  Inputs=+++
  Sum1 : Sum  Inputs=+++
  Switch : Switch  Criteria=u2 > Threshold
  Switch1 : Switch  Criteria=u2 > Threshold
  Terminator{1..7} (7 alike) : Terminator
  delay_estimation_1 : Constant  Value=comm_delay_estimation1
  delay_estimation_2 : Constant  Value=comm_delay_estimation2
  msg_decoding : Subsystem
  wires:
  Data Store Read/1 -> Equal/1
  Constant/1 -> Equal/2
  Bus Selector/8 -> Terminator7/1  "<Buffer_8>"
  Bus Selector/7 -> Terminator6/1  "<Buffer_7>"
  Switch/1 -> Bus Selector/1
  Bus Selector/1 -> msg_decoding/1(Msg_Temporal_Data)  "<Buffer_1>"
  Equal/1 -> Switch/2, [Rx_CAN1]
  Data Store Read1/1 -> Switch/1
  Data Store Read2/1 -> Switch/3
  "SET1 "/1 -> Data Store Write4/1
  msg_decoding/1(basic_cycle) -> Data Store Write2/1  "Rx_init_bc"
  msg_decoding/3(board_id) -> Cast1/1  "Rx_init_id"
  Constant3/1 -> Sum/2, Sum1/2
  Constant2/1 -> Multiply1/1
  Constant1/1 -> Multiply/1
  delay_estimation_2/1 -> Sum1/3
  Sum/1 -> Switch1/1
  msg_decoding/2(msg_count) -> Multiply/2, Multiply1/2  "Rx_init_mc"
  Multiply/1 -> Sum/1
  Multiply1/1 -> Sum1/1
  Sum1/1 -> Switch1/3
  delay_estimation_1/1 -> Sum/3
  [Rx_CAN1] -> Switch1/2
  Switch1/1 -> Cast/1
  Cast/1 -> Data Store Write1/1  "Rx_init_LT"
  Cast1/1 -> Data Store Write3/1
  Bus Selector/2 -> Terminator5/1  "<Buffer_2>"
  Bus Selector/3 -> Terminator2/1  "<Buffer_3>"
  Bus Selector/4 -> Terminator3/1  "<Buffer_4>"
  Bus Selector/5 -> Terminator4/1  "<Buffer_5>"
  Bus Selector/6 -> Terminator1/1  "<Buffer_6>"

== system HANcoder_E407_TTA_Group2/HANcoder STM32 Target - E407-STM32 algorithm/TTA CAN System/TTA System/Matrix Cycle Manager/Controller Matrix Cycle/Matrix_Cycle_Observation_DEBUG ==
  Data Store Read : DataStoreRead  DataStoreName=Master_ID
  Data Store Read1 : DataStoreRead  DataStoreName=Role_ID
  Data Store Read10 : DataStoreRead  DataStoreName=BC1_Sync_processed
  Data Store Read11 : DataStoreRead  DataStoreName=Sync_bc0_missed_counter
  Data Store Read12 : DataStoreRead  DataStoreName=Sync_bc1_missed_counter
  Data Store Read13 : DataStoreRead  DataStoreName=BC0_Vote4_processed
  Data Store Read14 : DataStoreRead  DataStoreName=Board4_error_counter
  Data Store Read2 : DataStoreRead  DataStoreName=BC0_Sync_processed
  Data Store Read3 : DataStoreRead  DataStoreName=Votes_count  DataStoreElements=Votes_count.First_Board#Votes_count.Second_Board#Votes_count.Third_Board
  Data Store Read4 : DataStoreRead  DataStoreName=Board1_error_counter
  Data Store Read5 : DataStoreRead  DataStoreName=Board2_error_counter
  Data Store Read6 : DataStoreRead  DataStoreName=Board3_error_counter
  Data Store Read7 : DataStoreRead  DataStoreName=BC0_Vote1_processed
  Data Store Read8 : DataStoreRead  DataStoreName=BC0_Vote2_processed
  Data Store Read9 : DataStoreRead  DataStoreName=BC0_Vote3_processed
  Terminator{,1..16} (17 alike) : Terminator
  wires:
  Data Store Read/1 -> Terminator1/1  "Master_ID_s"
  Data Store Read3/1 -> Terminator5/1  "votes_Board_1_DEBUG"
  Data Store Read3/2 -> Terminator6/1  "votes_Board_2_DEBUG"
  Data Store Read3/3 -> Terminator7/1  "votes_Board_3_DEBUG"
  Data Store Read4/1 -> Terminator8/1  "Board_1_error_counter_s"
  Data Store Read5/1 -> Terminator9/1  "Board_2_error_counter_s"
  Data Store Read6/1 -> Terminator10/1  "Board_3_error_counter_s"
  Data Store Read2/1 -> Terminator2/1  "BC0_sync_processed_s"
  Data Store Read7/1 -> Terminator3/1  "BC0_vote1_processed_s"
  Data Store Read8/1 -> Terminator4/1  "BC0_vote2_processed_s"
  Data Store Read9/1 -> Terminator11/1  "BC0_vote3_processed_s"
  Data Store Read10/1 -> Terminator12/1  "BC1_sync_processed_s"
  Data Store Read1/1 -> Terminator/1  "Role_ID_s"
  Data Store Read11/1 -> Terminator14/1  "sync_bc0_miss_counter_s"
  Data Store Read12/1 -> Terminator15/1  "sync_bc1_miss_counter_s"
  Data Store Read13/1 -> Terminator13/1  "BC0_vote4_processed_s"
  Data Store Read14/1 -> Terminator16/1  "Board_4_error_counter_s"
